simulink model "model"  (R2020a)
settings: Solver=FixedStepAuto  StartTime=0.0  StopTime=10.0  FixedStep=0.001  RelTol=1e-3
values from neighbouring files (symbols this model uses):
  Gss = ss(A,B,C,D)    [model_init.m]
undefined symbols (not defined in the file or in its folder): DiscIntNeverNeededParam
settings Model: Creator=Daniel  LastModifiedBy=Daniel

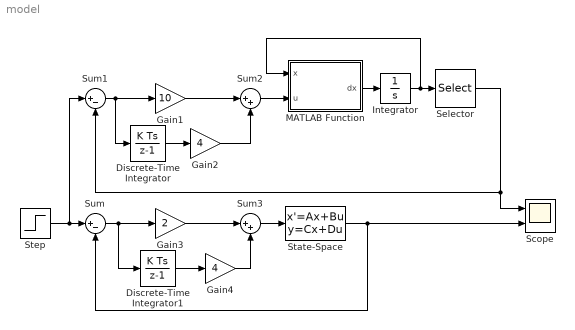
== system model ==
  Discrete-Time Integrator : DiscreteIntegrator  SampleTime=-1  ICPrevOutput=DiscIntNeverNeededParam  ICPrevScaledInput=DiscIntNeverNeededParam
  Discrete-Time Integrator1 : DiscreteIntegrator  SampleTime=-1  ICPrevOutput=DiscIntNeverNeededParam  ICPrevScaledInput=DiscIntNeverNeededParam
  Gain1 : Gain  Gain=10
  Gain2 : Gain  Gain=4
  Gain3 : Gain  Gain=2
  Gain4 : Gain  Gain=4
  Integrator : Integrator  InitialCondition=[0,0]
  MATLAB Function : MATLAB Function  TreatAsAtomicUnit=on
  Scope : Scope  NumInputPorts=2
  Selector : Selector  InputPortWidth=2  IndexOptions=Index vector (dialog)  Indices=2  OutputSizes=1
  State-Space : StateSpace  A=Gss.A  B=Gss.B  C=Gss.C  D=Gss.D  InitialCondition=0
  Step : Step  SampleTime=0
  Sum : Sum  Inputs=|+-
  Sum1 : Sum  Inputs=|+-
  Sum2 : Sum  Inputs=|++
  Sum3 : Sum  Inputs=|++
  wires:
  State-Space/1 -> Sum/2, Scope/2
  MATLAB Function/1(dx) -> Integrator/1
  Integrator/1 -> MATLAB Function/1(x), Selector/1
  Selector/1 -> Sum1/2, Scope/1
  Step/1 -> Sum/1, Sum1/1
  Sum1/1 -> Discrete-Time Integrator/1, Gain1/1
  Gain1/1 -> Sum2/1
  Sum2/1 -> MATLAB Function/2(u)
  Discrete-Time Integrator/1 -> Gain2/1
  Gain2/1 -> Sum2/2
  Gain4/1 -> Sum3/2
  Discrete-Time Integrator1/1 -> Gain4/1
  Gain3/1 -> Sum3/1
  Sum/1 -> Discrete-Time Integrator1/1, Gain3/1
  Sum3/1 -> State-Space/1

== matlab function model/MATLAB Function ==
  data: x input; u input; dx output
function dx = fcn(x,u)
    x1 = x(1);
    x2 = x(2);
    
    dx = zeros(2,1);
    
    dx(1) = -3*x1 - 1.5*x2 + u;
    dx(2) =  1*x1;
